simulink model "control_altura_probando"  (R2018b)
settings: Solver=VariableStepAuto  StartTime=0.0  StopTime=inf  RelTol=1e-3
undefined symbols (not defined in the file): Angular, Linear
libraries: robotlib x3
settings Model: Creator=luis  LastModifiedBy=luis
settings SFSimCC: SimUseLocalCustomCode=off
settings RTWCC: RTWUseLocalCustomCode=off

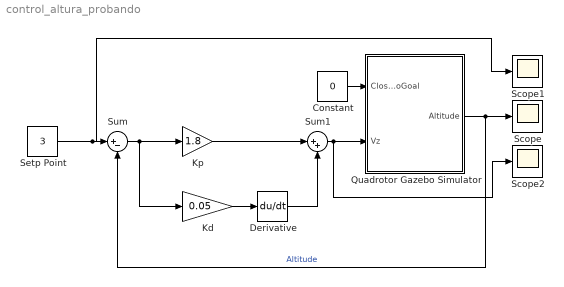
== system control_altura_probando ==
  Constant : Constant  Value=0
  Derivative : Derivative
  Kd : Gain  Gain=0.05
  Kp : Gain  Gain=1.8
  Quadrotor Gazebo Simulator : Subsystem
      mask Display: image('drone.jpeg');
  Scope : Scope
  Scope1 : Scope
  Scope2 : Scope
  Setp Point : Constant  Value=3
  Sum : Sum  Inputs=|+-
  Sum1 : Sum  Inputs=|++
  wires:
  Constant/1 -> Quadrotor Gazebo Simulator/1(CloseToGoal)
  Setp Point/1 -> Scope1/1, Sum/1
  Sum/1 -> Kd/1, Kp/1
  Derivative/1 -> Sum1/2
  Kp/1 -> Sum1/1
  Sum1/1 -> Scope2/1, Quadrotor Gazebo Simulator/2(Vz)
  Quadrotor Gazebo Simulator/1(Altitude) -> Scope/1, Sum/2  "Altitude"
  Kd/1 -> Derivative/1

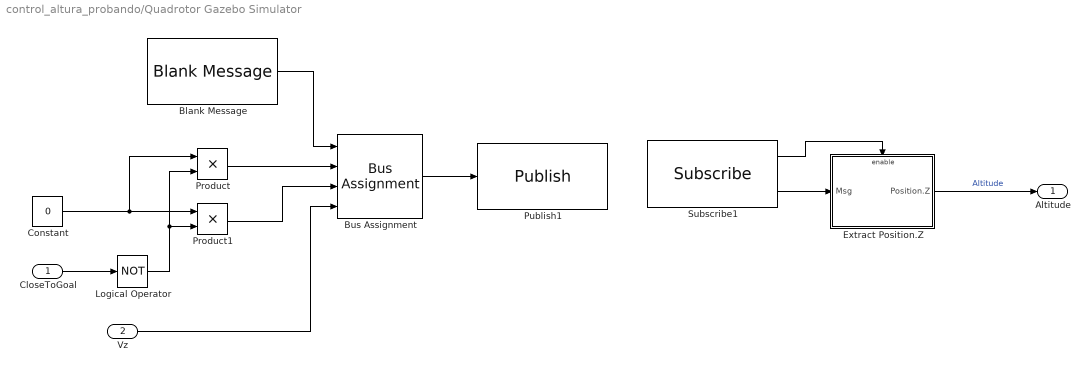
== system control_altura_probando/Quadrotor Gazebo Simulator ==
  CloseToGoal : Inport
  Vz : Inport  Port=2
  Blank Message : robotlib/Blank Message  messageClass=Message  entityType=geometry_msgs/Twist  messageType=geometry_msgs/Twist  SampleTime=-1
      settings: SourceProductBaseCode=RO
  Bus Assignment : BusAssignment  DialogController=Simulink.DDGSource_BusAssignment  AssignedSignals=Linear.X,Angular.Z,Linear.Z
  Constant : Constant  Value=0
  Extract Position.Z : Subsystem
  Logical Operator : Logic  Operator=NOT  AllPortsSameDT=off  OutDataTypeStr=boolean
  Product : Product
  Product1 : Product
  Publish1 : robotlib/Publish  topicSource=Select from ROS network  topic=/quadrotor_1/cmd_vel  messageType=geometry_msgs/Twist  messageQueueLength=105
      settings: SourceProductBaseCode=RO
  Subscribe1 : robotlib/Subscribe  topicSource=Select from ROS network  topic=/quadrotor_1/ground_truth/state  messageType=nav_msgs/Odometry  sampleTime=-1  messageQueueLength=51
      settings: SourceProductBaseCode=RO
  Altitude : Outport
  wires:
  Bus Assignment/1 -> Publish1/1
  Blank Message/1 -> Bus Assignment/1
  Logical Operator/1 -> Product1/2, Product/2
  Product1/1 -> Bus Assignment/3
  CloseToGoal/1 -> Logical Operator/1
  Product/1 -> Bus Assignment/2
  Constant/1 -> Product/1, Product1/1
  Vz/1 -> Bus Assignment/4
  Subscribe1/2 -> Extract Position.Z/1(Msg)
  Subscribe1/1 -> Extract Position.Z/Enable
  Extract Position.Z/1(Position.Z) -> Altitude/1  "Altitude"

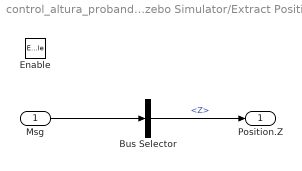
== system control_altura_probando/Quadrotor Gazebo Simulator/Extract Position.Z ==
  Msg : Inport
  Enable : EnablePort
  Bus Selector : BusSelector  OutputSignals=Pose.Pose.Position.Z
  Position.Z : Outport
  wires:
  Msg/1 -> Bus Selector/1
  Bus Selector/1 -> Position.Z/1  "<Z>"
